simulink model "Lab1_4_2_sol"  (R2023a)
settings: Solver=ode45  StartTime=0.0  StopTime=10000/20e6  RelTol=1e-3  EnableMultiTasking=on
undefined symbols (not defined in the file): MyCoeffs, xc7k325tfbg676
libraries: hdlBasic x97, dspfdesign x1, hdlUtilities x1, vmcUtilities x1
settings Model: Creator=danielm  LastModifiedBy=robg
settings SolverCC: AlgebraicLoopSolver=TrustRegion
settings DataIOCC: LimitDataPoints=on  SaveFormat=Array  ReturnWorkspaceOutputs=off
settings OptimizationCC: LifeSpan=inf
settings DebuggingCC: UnderspecifiedInitializationDetection=Classic  MergeDetectMultiDrivingBlocksExec=none  SolverPrmCheckMsg=warning  UnconnectedInputMsg=warning  UnconnectedOutputMsg=warning  UnconnectedLineMsg=warning  SFUnexpectedBacktrackingDiag=warning  SFNoUnconditionalDefaultTransitionDiag=warning  ArithmeticOperatorsInVariantConditions=warning
settings HardwareCC: ProdBitPerPointer=32  ProdBitPerSizeT=32  ProdBitPerPtrDiffT=32  ProdLargestAtomicFloat=None  ProdIntDivRoundTo=Undefined  ProdEndianess=Unspecified  ProdWordSize=32  ProdHWDeviceType=32-bit Generic
settings ModelReferenceCC: EnableRefExpFcnMdlSchedulingChecks=on  PropagateSignalLabelsOutOfModel=off
settings SFSimCC: SimUseLocalCustomCode=off  CustomCodeUndefinedFunction=UseInterfaceOnly
settings RTWCC: RTWUseLocalCustomCode=off  DLArmComputeVersion=19.05
settings CodeAppCC: StateflowObjectComments=on
settings GRTTargetCC: TargetLangStandard=C89/C90 (ANSI)
settings ConfigComp: CovMetricSettings=dw  CovSaveCumulativeToWorkspaceVar=on  CovSaveSingleToWorkspaceVar=on  CovExternalEMLEnable=off  CovSFcnEnable=off

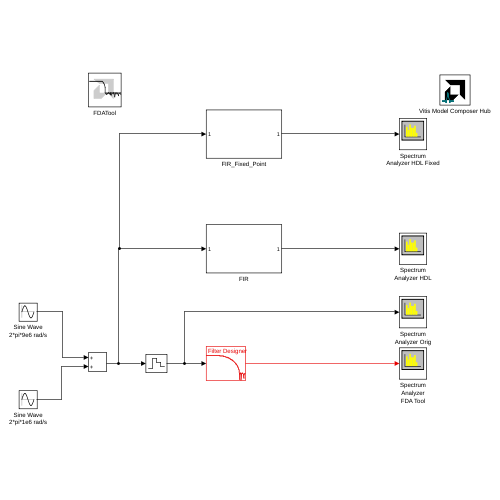
[thumbnail: Simulink's stored preview of the top-level diagram]
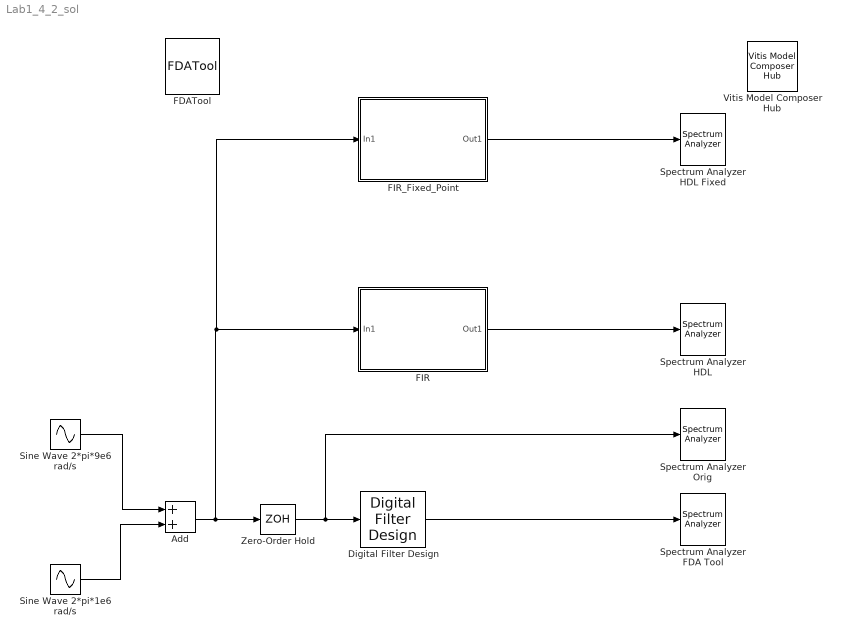
== system Lab1_4_2_sol ==
  Add : Sum
  Digital Filter Design : dspfdesign/Digital Filter Design  mwdsp_browser_bugfix_var=off
  FDATool : hdlUtilities/FDATool  block_type=fdatool
      settings: infoedit=FDATool
  FIR : Subsystem
  FIR_Fixed_Point : Subsystem
  Sine Wave 2*pi*1e6 rad/s : Sin  Frequency=2*pi*1e6  SampleTime=0
  Sine Wave 2*pi*9e6 rad/s : Sin  Frequency=2*pi*9e6  SampleTime=0
  Spectrum Analyzer FDA Tool : SpectrumAnalyzer  WindowPosition=[481 213 576 420]  Method=Welch  SampleRate=20000000  AveragingMethod=Exponential  YLimits=[-187.0838,47.1991]  ChannelNames="[\"\"]"  DefaultConfigurationName=spbscopes.SpectrumAnalyzerBlockCfg
  Spectrum Analyzer HDL : SpectrumAnalyzer  WindowPosition=[489 221 560 420]  Method=Welch  SampleRate=20000000  AveragingMethod=Exponential  YLimits=[-196.4873,48.2439]  ChannelNames="[\"\"]"  DefaultConfigurationName=spbscopes.SpectrumAnalyzerBlockCfg
  Spectrum Analyzer HDL Fixed : SpectrumAnalyzer  WindowPosition=[485 217 568 420]  Method=Welch  SampleRate=20000000  AveragingMethod=Exponential  YLimits=[-196.7604,54.964]  ChannelNames="[\"\"]"  DefaultConfigurationName=spbscopes.SpectrumAnalyzerBlockCfg
  Spectrum Analyzer Orig : SpectrumAnalyzer  WindowPosition=[485 217 568 420]  Method=Welch  SampleRate=20000000  AveragingMethod=Exponential  YLimits=[-153.2838,43.4257]  ChannelNames="[\"\"]"  DefaultConfigurationName=spbscopes.SpectrumAnalyzerBlockCfg
  Vitis Model Composer Hub : vmcUtilities/Vitis Model Composer Hub  Tag=genX  CodeGeneration=off  StartColumn=1  NumberOfColumns=1  TargetDirectory=./code  exportDesign=off  analyzeDesign=off  validateDesignOnHw=off  ExportType=System Generator  IpVendor=xilinx.com  IpLibrary=hls  IpVersion=1.0  IpHWLanguage=Verilog  AieCompilerOptions={}  AieSimulatorOptions={}  CreateTestbench=off  TestbenchStackSize=10  RunRtlSim=off  RunCSim=off  RunAieSim=off  AieSimTimeout=50000  RunAieSimProfiling=off  LaunchVitisAnalyzer=off  PlotOutput=off  RunX86Sim=off  X86SimTimeout=10  GenHwImage=off  GenLibadfXo=off  GenHwValidationCode=off  PlatformType=Not Specified  HwSystemType=Baremetal  HwValidationTarget=hw  ProjDevice=xc7k325tfbg676-3  ProjDevicePart=xc7k325tfbg676-3  SamplePeriod=-1  ClockFrequency=200  DataPathParallelism=1  xilinxfamily=kintex7  part=xc7k325t  speed=-3  package=fbg676  directory=./netlist_part2  testbench=off  incr_netlist=off  synthesis_tool=Vivado  clock_wrapper=Clock Enables  dbl_ovrd=According to Block Masks  dcm_input_clock_period=10  sysclk_period=50  simulink_period=1/20e6  eval_field=0  IPInfoJsonString="{\"HDLSubsystem\":{\"SubsystemName\":\"FIR_Fixed_Point\",\"IPName\":\"FIR_Fixed_Point\",\"IPLibrary\":\"VMC\",\"IPVendor\":\"User Company\",\"IPVersion\":\"1.0\"}}"  LogFileName=''  NThreads=4
  Zero-Order Hold : ZeroOrderHold  SampleTime=1/20e6
  wires:
  Sine Wave 2*pi*9e6 rad/s/1 -> Add/1
  Sine Wave 2*pi*1e6 rad/s/1 -> Add/2
  Digital Filter Design/1 -> Spectrum Analyzer FDA Tool/1
  Zero-Order Hold/1 -> Spectrum Analyzer Orig/1, Digital Filter Design/1
  Add/1 -> FIR/1(In1), FIR_Fixed_Point/1(In1), Zero-Order Hold/1
  FIR/1(Out1) -> Spectrum Analyzer HDL/1
  FIR_Fixed_Point/1(Out1) -> Spectrum Analyzer HDL Fixed/1

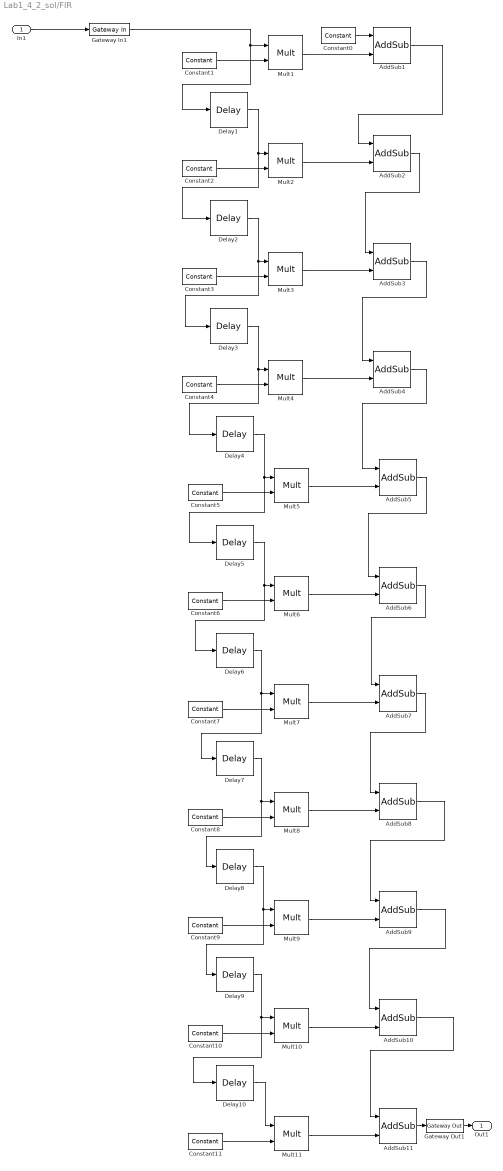
== system Lab1_4_2_sol/FIR ==
  In1 : Inport
  AddSub{1..11} (11 alike) : hdlBasic/AddSub  mode=Addition  use_carryin=off  use_carryout=off  en=off  latency=1  precision=Full  arith_type=Unsigned  n_bits=16  bin_pt=14  quantization=Truncate  overflow=Wrap  use_behavioral_HDL=off  hw_selection=Fabric  pipelined=off  XmcBlockStatus=1  maskContainerNames=tabcontainer1  block_type=addsub  block_config=sysgen:Addsub_config
  Constant0 : hdlBasic/Constant  const=0  gui_display_data_type=Floating-point  arith_type=Floating-point  n_bits=16  bin_pt=14  preci_type=Single  exp_width=8  frac_width=24  explicit_period=off  period=1  XmcBlockStatus=1  maskContainerNames=tabcontainer1  block_type=constant  block_config=sysgen:Constant_config
  "Constant1 " : hdlBasic/Constant  const=MyCoeffs(1)  gui_display_data_type=Floating-point  arith_type=Floating-point  n_bits=16  bin_pt=14  preci_type=Single  exp_width=8  frac_width=24  explicit_period=on  period=1/20e6  XmcBlockStatus=1  maskContainerNames=tabcontainer1  block_type=constant  block_config=sysgen:Constant_config
  Constant10 : hdlBasic/Constant  const=MyCoeffs(10)  gui_display_data_type=Floating-point  arith_type=Floating-point  n_bits=16  bin_pt=14  preci_type=Single  exp_width=8  frac_width=24  explicit_period=on  period=1/20e6  XmcBlockStatus=1  maskContainerNames=tabcontainer1  block_type=constant  block_config=sysgen:Constant_config
  Constant11 : hdlBasic/Constant  const=MyCoeffs(11)  gui_display_data_type=Floating-point  arith_type=Floating-point  n_bits=16  bin_pt=14  preci_type=Single  exp_width=8  frac_width=24  explicit_period=on  period=1/20e6  XmcBlockStatus=1  maskContainerNames=tabcontainer1  block_type=constant  block_config=sysgen:Constant_config
  "Constant2 " : hdlBasic/Constant  const=MyCoeffs(2)  gui_display_data_type=Floating-point  arith_type=Floating-point  n_bits=16  bin_pt=14  preci_type=Single  exp_width=8  frac_width=24  explicit_period=on  period=1/20e6  XmcBlockStatus=1  maskContainerNames=tabcontainer1  block_type=constant  block_config=sysgen:Constant_config
  Constant3 : hdlBasic/Constant  const=MyCoeffs(3)  gui_display_data_type=Floating-point  arith_type=Floating-point  n_bits=16  bin_pt=14  preci_type=Single  exp_width=8  frac_width=24  explicit_period=on  period=1/20e6  XmcBlockStatus=1  maskContainerNames=tabcontainer1  block_type=constant  block_config=sysgen:Constant_config
  Constant4 : hdlBasic/Constant  const=MyCoeffs(4)  gui_display_data_type=Floating-point  arith_type=Floating-point  n_bits=16  bin_pt=14  preci_type=Single  exp_width=8  frac_width=24  explicit_period=on  period=1/20e6  XmcBlockStatus=1  maskContainerNames=tabcontainer1  block_type=constant  block_config=sysgen:Constant_config
  Constant5 : hdlBasic/Constant  const=MyCoeffs(5)  gui_display_data_type=Floating-point  arith_type=Floating-point  n_bits=16  bin_pt=14  preci_type=Single  exp_width=8  frac_width=24  explicit_period=on  period=1/20e6  XmcBlockStatus=1  maskContainerNames=tabcontainer1  block_type=constant  block_config=sysgen:Constant_config
  Constant6 : hdlBasic/Constant  const=MyCoeffs(6)  gui_display_data_type=Floating-point  arith_type=Floating-point  n_bits=16  bin_pt=14  preci_type=Single  exp_width=8  frac_width=24  explicit_period=on  period=1/20e6  XmcBlockStatus=1  maskContainerNames=tabcontainer1  block_type=constant  block_config=sysgen:Constant_config
  Constant7 : hdlBasic/Constant  const=MyCoeffs(7)  gui_display_data_type=Floating-point  arith_type=Floating-point  n_bits=16  bin_pt=14  preci_type=Single  exp_width=8  frac_width=24  explicit_period=on  period=1/20e6  XmcBlockStatus=1  maskContainerNames=tabcontainer1  block_type=constant  block_config=sysgen:Constant_config
  Constant8 : hdlBasic/Constant  const=MyCoeffs(8)  gui_display_data_type=Floating-point  arith_type=Floating-point  n_bits=16  bin_pt=14  preci_type=Single  exp_width=8  frac_width=24  explicit_period=on  period=1/20e6  XmcBlockStatus=1  maskContainerNames=tabcontainer1  block_type=constant  block_config=sysgen:Constant_config
  Constant9 : hdlBasic/Constant  const=MyCoeffs(9)  gui_display_data_type=Floating-point  arith_type=Floating-point  n_bits=16  bin_pt=14  preci_type=Single  exp_width=8  frac_width=24  explicit_period=on  period=1/20e6  XmcBlockStatus=1  maskContainerNames=tabcontainer1  block_type=constant  block_config=sysgen:Constant_config
  Delay{1..10} (10 alike) : hdlBasic/Delay  rst=off  en=off  latency=2  reg_retiming=off  XmcBlockStatus=1  maskContainerNames=group1  block_type=delay  block_config=sysgen:Delay_config
  Gateway In1 : hdlBasic/Gateway In  gui_display_data_type=Floating-point  arith_type=Floating-point  n_bits=16  bin_pt=14  preci_type=Single  exp_width=8  frac_width=24  rows=1  columns=1  quantization="Round  (unbiased: +/- Inf)"  overflow=Saturate  period=1/20e6  UseAsADC=off  ADCChannel='1'  interface=None  automatic_assignment=on  address_offset=hex2dec('00')  intf_name=''  intf_description=''  default_value=0  timing_constraint=None  locs_specified=off  LOCs={}  io_standard={}  inherit_from_input=off  hdl_port=on  XmcBlockStatus=1  maskContainerNames=group4  block_type=gatewayin  block_config=sysgen:gateway_in_config  block_width_w=590  block_height_w=620  block_width=640  block_height=850
  Gateway Out1 : hdlBasic/Gateway Out  inherit_from_input=off  hdl_port=on  rows=1  columns=1  UseAsDAC=off  DACChannel='1'  interface=None  automatic_assignment=on  address_offset=hex2dec('00')  intf_name=''  intf_description=''  timing_constraint=None  locs_specified=off  LOCs={}  io_standard={}  XmcBlockStatus=1  maskContainerNames=group4  block_type=gatewayout  block_config=sysgen:gateway_out_config  block_width_w=590  block_height_w=620  block_width=620  block_height=750
  Mult{1..11} (11 alike) : hdlBasic/Mult  precision=Full  arith_type="Signed  (2's comp)"  n_bits=16  bin_pt=14  quantization=Truncate  overflow=Wrap  en=off  latency=3  opt_float=off  fp_mult_usage=No Usage  use_behavioral_HDL=off  opt=Speed  use_embedded=on  optimum_pipeline=off  pipeline=on  use_rpm=on  placement_style=Triangular  XmcBlockStatus=1  maskContainerNames=group1  block_type=mult  block_config=sysgen:Mult_config  block_width=598  block_height=876
  Out1 : Outport  VectorParamsAs1DForOutWhenUnconnected=off
  wires:
  "Constant1 "/1 -> Mult1/2
  Mult1/1 -> AddSub1/2
  Gateway In1/1 -> Delay1/1, Mult1/1
  Constant0/1 -> AddSub1/1
  "Constant2 "/1 -> Mult2/2
  Mult2/1 -> AddSub2/2
  Delay1/1 -> Mult2/1, Delay2/1
  Constant3/1 -> Mult3/2
  Mult3/1 -> AddSub3/2
  AddSub2/1 -> AddSub3/1
  Delay2/1 -> Delay3/1, Mult3/1
  Constant4/1 -> Mult4/2
  Mult4/1 -> AddSub4/2
  Delay3/1 -> Mult4/1, Delay4/1
  Constant5/1 -> Mult5/2
  Mult5/1 -> AddSub5/2
  AddSub5/1 -> AddSub6/1
  Delay4/1 -> Mult5/1, Delay5/1
  Constant6/1 -> Mult6/2
  Mult6/1 -> AddSub6/2
  Delay5/1 -> Mult6/1, Delay6/1
  Constant7/1 -> Mult7/2
  Mult7/1 -> AddSub7/2
  Delay6/1 -> Mult7/1, Delay7/1
  Constant8/1 -> Mult8/2
  Mult8/1 -> AddSub8/2
  AddSub7/1 -> AddSub8/1
  Delay7/1 -> Mult8/1, Delay8/1
  Constant9/1 -> Mult9/2
  Mult9/1 -> AddSub9/2
  AddSub8/1 -> AddSub9/1
  Delay8/1 -> Mult9/1, Delay9/1
  Constant10/1 -> Mult10/2
  Mult10/1 -> AddSub10/2
  AddSub9/1 -> AddSub10/1
  Delay9/1 -> Mult10/1, Delay10/1
  Constant11/1 -> Mult11/2
  Mult11/1 -> AddSub11/2
  Delay10/1 -> Mult11/1
  AddSub3/1 -> AddSub4/1
  AddSub4/1 -> AddSub5/1
  AddSub6/1 -> AddSub7/1
  AddSub10/1 -> AddSub11/1
  AddSub1/1 -> AddSub2/1
  In1/1 -> Gateway In1/1
  AddSub11/1 -> Gateway Out1/1
  Gateway Out1/1 -> Out1/1

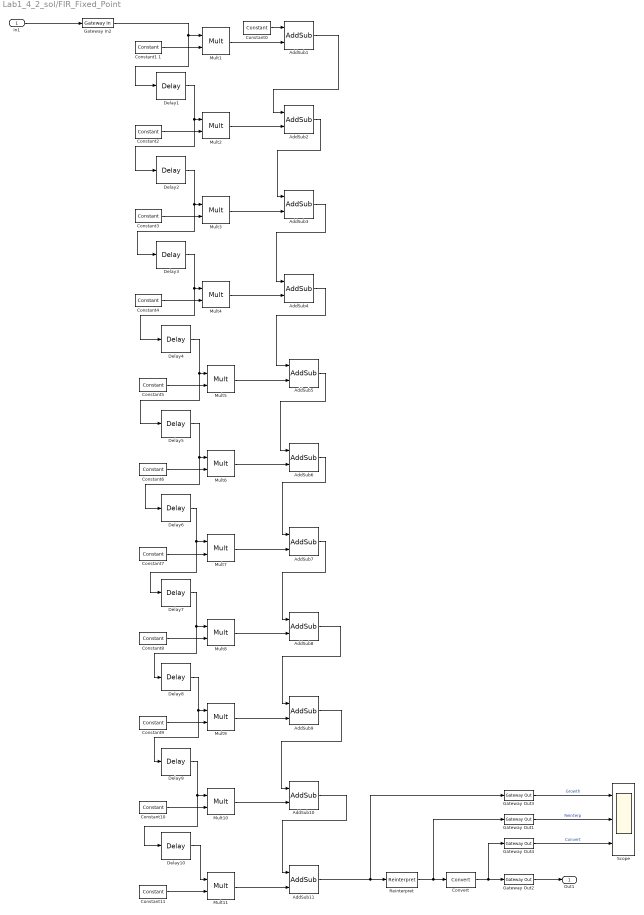
== system Lab1_4_2_sol/FIR_Fixed_Point ==
  In1 : Inport
  AddSub{1..11} (11 alike) : hdlBasic/AddSub  mode=Addition  use_carryin=off  use_carryout=off  en=off  latency=1  precision=Full  arith_type=Unsigned  n_bits=16  bin_pt=14  quantization=Truncate  overflow=Wrap  use_behavioral_HDL=off  hw_selection=Fabric  pipelined=off  XmcBlockStatus=1  maskContainerNames=tabcontainer1  block_type=addsub  block_config=sysgen:Addsub_config
  Constant0 : hdlBasic/Constant  const=0  gui_display_data_type=Fixed-point  arith_type=Signed (2's comp)  n_bits=16  bin_pt=14  preci_type=Single  exp_width=8  frac_width=24  explicit_period=off  period=1  XmcBlockStatus=1  maskContainerNames=tabcontainer1  block_type=constant  block_config=sysgen:Constant_config
  Constant1 1 : hdlBasic/Constant  const=MyCoeffs(1)  gui_display_data_type=Fixed-point  arith_type=Signed (2's comp)  n_bits=16  bin_pt=14  preci_type=Single  exp_width=8  frac_width=24  explicit_period=off  period=1/20e6  XmcBlockStatus=1  maskContainerNames=tabcontainer1  block_type=constant  block_config=sysgen:Constant_config
  Constant10 : hdlBasic/Constant  const=MyCoeffs(10)  gui_display_data_type=Fixed-point  arith_type=Signed (2's comp)  n_bits=16  bin_pt=14  preci_type=Single  exp_width=8  frac_width=24  explicit_period=on  period=1/20e6  XmcBlockStatus=1  maskContainerNames=tabcontainer1  block_type=constant  block_config=sysgen:Constant_config
  Constant11 : hdlBasic/Constant  const=MyCoeffs(11)  gui_display_data_type=Fixed-point  arith_type=Signed (2's comp)  n_bits=16  bin_pt=14  preci_type=Single  exp_width=8  frac_width=24  explicit_period=on  period=1/20e6  XmcBlockStatus=1  maskContainerNames=tabcontainer1  block_type=constant  block_config=sysgen:Constant_config
  "Constant2 " : hdlBasic/Constant  const=MyCoeffs(2)  gui_display_data_type=Fixed-point  arith_type=Signed (2's comp)  n_bits=16  bin_pt=14  preci_type=Single  exp_width=8  frac_width=24  explicit_period=on  period=1/20e6  XmcBlockStatus=1  maskContainerNames=tabcontainer1  block_type=constant  block_config=sysgen:Constant_config
  Constant3 : hdlBasic/Constant  const=MyCoeffs(3)  gui_display_data_type=Fixed-point  arith_type=Signed (2's comp)  n_bits=16  bin_pt=14  preci_type=Single  exp_width=8  frac_width=24  explicit_period=on  period=1/20e6  XmcBlockStatus=1  maskContainerNames=tabcontainer1  block_type=constant  block_config=sysgen:Constant_config
  Constant4 : hdlBasic/Constant  const=MyCoeffs(4)  gui_display_data_type=Fixed-point  arith_type=Signed (2's comp)  n_bits=16  bin_pt=14  preci_type=Single  exp_width=8  frac_width=24  explicit_period=on  period=1/20e6  XmcBlockStatus=1  maskContainerNames=tabcontainer1  block_type=constant  block_config=sysgen:Constant_config
  Constant5 : hdlBasic/Constant  const=MyCoeffs(5)  gui_display_data_type=Fixed-point  arith_type=Signed (2's comp)  n_bits=16  bin_pt=14  preci_type=Single  exp_width=8  frac_width=24  explicit_period=on  period=1/20e6  XmcBlockStatus=1  maskContainerNames=tabcontainer1  block_type=constant  block_config=sysgen:Constant_config
  Constant6 : hdlBasic/Constant  const=MyCoeffs(6)  gui_display_data_type=Fixed-point  arith_type=Signed (2's comp)  n_bits=16  bin_pt=14  preci_type=Single  exp_width=8  frac_width=24  explicit_period=on  period=1/20e6  XmcBlockStatus=1  maskContainerNames=tabcontainer1  block_type=constant  block_config=sysgen:Constant_config
  Constant7 : hdlBasic/Constant  const=MyCoeffs(7)  gui_display_data_type=Fixed-point  arith_type=Signed (2's comp)  n_bits=16  bin_pt=14  preci_type=Single  exp_width=8  frac_width=24  explicit_period=on  period=1/20e6  XmcBlockStatus=1  maskContainerNames=tabcontainer1  block_type=constant  block_config=sysgen:Constant_config
  Constant8 : hdlBasic/Constant  const=MyCoeffs(8)  gui_display_data_type=Fixed-point  arith_type=Signed (2's comp)  n_bits=16  bin_pt=14  preci_type=Single  exp_width=8  frac_width=24  explicit_period=on  period=1/20e6  XmcBlockStatus=1  maskContainerNames=tabcontainer1  block_type=constant  block_config=sysgen:Constant_config
  Constant9 : hdlBasic/Constant  const=MyCoeffs(9)  gui_display_data_type=Fixed-point  arith_type=Signed (2's comp)  n_bits=16  bin_pt=14  preci_type=Single  exp_width=8  frac_width=24  explicit_period=on  period=1/20e6  XmcBlockStatus=1  maskContainerNames=tabcontainer1  block_type=constant  block_config=sysgen:Constant_config
  Convert : hdlBasic/Convert  gui_display_data_type=Fixed-point  arith_type=Signed (2's comp)  n_bits=16  bin_pt=13  float_type=Single  exp_bits=8  fraction_bits=24  quantization=Truncate  overflow=Wrap  en=off  latency=1  pipeline=off  XmcBlockStatus=1  maskContainerNames=group2  block_type=convert  block_config=sysgen:Convert_config  block_width=595  block_height=885
  Delay{1..10} (10 alike) : hdlBasic/Delay  rst=off  en=off  latency=2  reg_retiming=off  XmcBlockStatus=1  maskContainerNames=group1  block_type=delay  block_config=sysgen:Delay_config
  Gateway In2 : hdlBasic/Gateway In  gui_display_data_type=Fixed-point  arith_type=Signed (2's comp)  n_bits=16  bin_pt=14  preci_type=Single  exp_width=8  frac_width=24  rows=1  columns=1  quantization="Round  (unbiased: +/- Inf)"  overflow=Saturate  period=1/20e6  UseAsADC=off  ADCChannel='1'  interface=None  automatic_assignment=on  address_offset=hex2dec('00')  intf_name=''  intf_description=''  default_value=0  timing_constraint=None  locs_specified=off  LOCs={}  io_standard={}  inherit_from_input=off  hdl_port=on  XmcBlockStatus=1  maskContainerNames=group4  block_type=gatewayin  block_config=sysgen:gateway_in_config  block_width_w=590  block_height_w=620  block_width=640  block_height=850
  Gateway Out{1..4} (4 alike) : hdlBasic/Gateway Out  inherit_from_input=off  hdl_port=on  rows=1  columns=1  UseAsDAC=off  DACChannel='1'  interface=None  automatic_assignment=on  address_offset=hex2dec('00')  intf_name=''  intf_description=''  timing_constraint=None  locs_specified=off  LOCs={}  io_standard={}  XmcBlockStatus=1  maskContainerNames=group4  block_type=gatewayout  block_config=sysgen:gateway_out_config  block_width_w=590  block_height_w=620  block_width=620  block_height=750
  Mult{1..11} (11 alike) : hdlBasic/Mult  precision=Full  arith_type="Signed  (2's comp)"  n_bits=16  bin_pt=14  quantization=Truncate  overflow=Wrap  en=off  latency=3  opt_float=off  fp_mult_usage=No Usage  use_behavioral_HDL=off  opt=Speed  use_embedded=on  optimum_pipeline=off  pipeline=on  use_rpm=on  placement_style=Triangular  XmcBlockStatus=1  maskContainerNames=group1  block_type=mult  block_config=sysgen:Mult_config  block_width=598  block_height=876
  Reinterpret : hdlBasic/Reinterpret  force_arith_type=off  arith_type=Unsigned  force_bin_pt=on  bin_pt=27  XmcBlockStatus=1  maskContainerNames=group1  block_type=reinterpret  block_config=sysgen:Reinterpret_config
  Scope : Scope  NumInputPorts=3
  Out1 : Outport  VectorParamsAs1DForOutWhenUnconnected=off
  wires:
  Mult1/1 -> AddSub1/2
  Gateway In2/1 -> Delay1/1, Mult1/1
  Constant0/1 -> AddSub1/1
  "Constant2 "/1 -> Mult2/2
  Mult2/1 -> AddSub2/2
  Delay1/1 -> Mult2/1, Delay2/1
  Constant3/1 -> Mult3/2
  Mult3/1 -> AddSub3/2
  AddSub2/1 -> AddSub3/1
  Delay2/1 -> Delay3/1, Mult3/1
  Constant4/1 -> Mult4/2
  Mult4/1 -> AddSub4/2
  Delay3/1 -> Mult4/1, Delay4/1
  Constant5/1 -> Mult5/2
  Mult5/1 -> AddSub5/2
  AddSub5/1 -> AddSub6/1
  Delay4/1 -> Mult5/1, Delay5/1
  Constant6/1 -> Mult6/2
  Mult6/1 -> AddSub6/2
  Delay5/1 -> Mult6/1, Delay6/1
  Constant7/1 -> Mult7/2
  Mult7/1 -> AddSub7/2
  Delay6/1 -> Mult7/1, Delay7/1
  Constant8/1 -> Mult8/2
  Mult8/1 -> AddSub8/2
  AddSub7/1 -> AddSub8/1
  Delay7/1 -> Mult8/1, Delay8/1
  Constant9/1 -> Mult9/2
  Mult9/1 -> AddSub9/2
  AddSub8/1 -> AddSub9/1
  Delay8/1 -> Mult9/1, Delay9/1
  Constant10/1 -> Mult10/2
  Mult10/1 -> AddSub10/2
  AddSub9/1 -> AddSub10/1
  Delay9/1 -> Mult10/1, Delay10/1
  Constant11/1 -> Mult11/2
  Mult11/1 -> AddSub11/2
  Delay10/1 -> Mult11/1
  AddSub3/1 -> AddSub4/1
  AddSub4/1 -> AddSub5/1
  AddSub6/1 -> AddSub7/1
  AddSub10/1 -> AddSub11/1
  AddSub1/1 -> AddSub2/1
  Constant1 1/1 -> Mult1/2
  In1/1 -> Gateway In2/1
  AddSub11/1 -> Gateway Out3/1, Reinterpret/1
  Gateway Out2/1 -> Out1/1
  Reinterpret/1 -> Gateway Out1/1, Convert/1
  Convert/1 -> Gateway Out4/1, Gateway Out2/1
  Gateway Out3/1 -> Scope/1  "Growth"
  Gateway Out1/1 -> Scope/2  "Reinterp"
  Gateway Out4/1 -> Scope/3  "Convert"
